simulink model "test1"  (R2014a)
settings: Solver=ode1  StartTime=0.0  StopTime=inf  FixedStep=0.01  RelTol=1e-3
settings Model: ExtModeTrigDuration=5000  Creator=sasson  LastModifiedBy=sasson
settings SolverCC: PositivePriorityOrder=on
settings HardwareCC: ProdIntDivRoundTo=Zero  ProdEndianess=LittleEndian  ProdHWDeviceType=Generic->32-bit x86 compatible
settings RTWCC: SystemTargetFile=rtwin.tlc  TemplateMakefile=rtwin.tmf  Description=Real-Time Windows Target  ProcessScript=rtwin_make_rtw_hook  TargetLang=C++
settings CodeAppCC: MaxIdLength=95
settings RTWinTargetCC: TargetLibSuffix=_rtwin.lib  TargetPreCompLibLocation=C:\Program Files\MATLAB\R2014a\toolbox\rtw\targets\rtwin\lib\win64

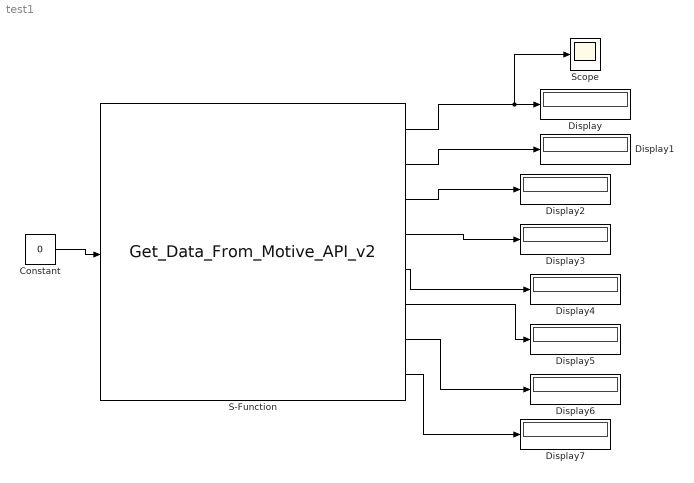
== system test1 ==
  Constant : Constant  Value=0
  Display{,1..7} (8 alike) : Display
  S-Function : S-Function  FunctionName=Get_Data_From_Motive_API_v2  EnableBusSupport=off
  Scope : Scope
      settings: YMin=0  YMax=0.15
  wires:
  Constant/1 -> S-Function/1
  S-Function/1 -> Scope/1, Display/1
  S-Function/2 -> Display1/1
  S-Function/3 -> Display2/1
  S-Function/4 -> Display3/1
  S-Function/5 -> Display4/1
  S-Function/6 -> Display5/1
  S-Function/7 -> Display6/1
  S-Function/8 -> Display7/1
